simulink model "plant_model_exercise"  (R2023b)
settings: Solver=VariableStepAuto  StartTime=0.0  StopTime=10.0  RelTol=1e-3
InitFcn:
  | Tstall = 20;
  | NoLoadSpeed = 20;
  | J_inertia = 1;
  | b_damping = 0;
  | load('MyTest.mat')
  | Vn = 30;
  | wNL = NoLoadSpeed;
  | K = Vn/wNL;
  | R = Vn^2/wNL/Tstall;
  | L = 1e-5;
settings Model: Creator=Harish  LastModifiedBy=Harish

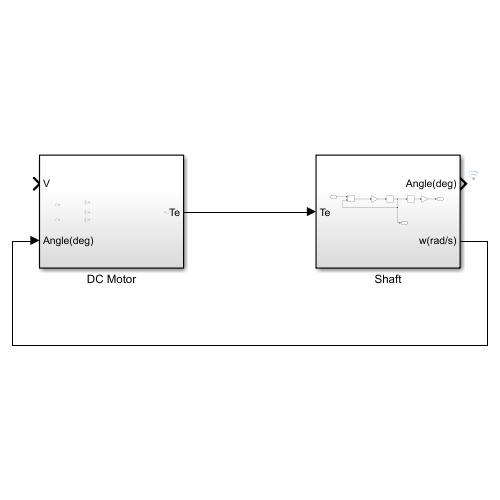
[thumbnail: Simulink's stored preview of the top-level diagram]
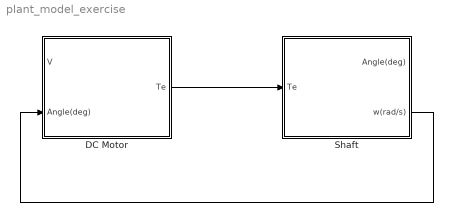
== system plant_model_exercise ==
  DC Motor : Subsystem
  Shaft : Subsystem
  wires:
  Shaft/2(w(rad/s)) -> DC Motor/2(Angle(deg))
  DC Motor/1(Te) -> Shaft/1(Te)

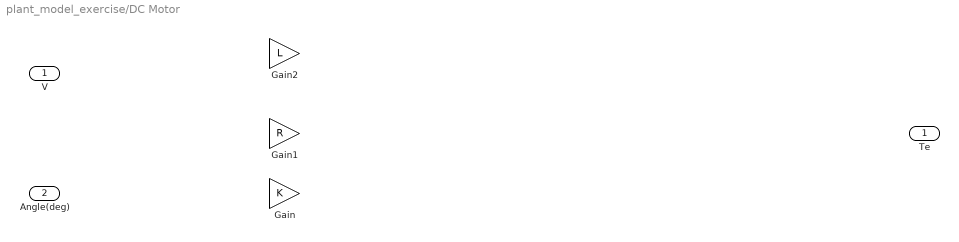
== system plant_model_exercise/DC Motor ==
  V : Inport
  Angle(deg) : Inport  Port=2
  Gain : Gain  Gain=K
  Gain1 : Gain  Gain=R
  Gain2 : Gain  Gain=L
  Te : Outport

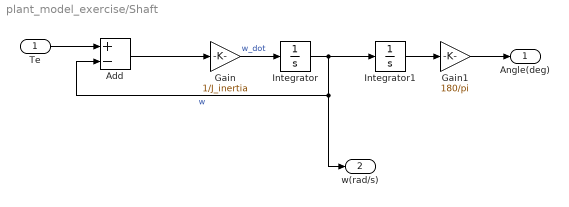
== system plant_model_exercise/Shaft ==
  Te : Inport
  Add : Sum  Inputs=+-
  Gain : Gain  Gain=1/J_inertia
  Gain1 : Gain  Gain=180/pi
  Integrator : Integrator
  Integrator1 : Integrator
  Angle(deg) : Outport
  w(rad/s) : Outport  Port=2
  wires:
  Te/1 -> Add/1
  Gain/1 -> Integrator/1  "w_dot"
  Integrator/1 -> Integrator1/1, Add/2, w(rad/s)/1  "w"
  Integrator1/1 -> Gain1/1
  Gain1/1 -> Angle(deg)/1
  Add/1 -> Gain/1
